simulink model "FreqSweep_HIL"  (Simulink 7.0)
settings: Solver=FixedStepDiscrete  SolverMode=SingleTasking  StartTime=0.0  StopTime=137*20*8*4  FixedStep=1  RelTol=1e-3
InitFcn:
  | %% DSPBuilder Start
  | alt_dspbuilder_update_model(bdroot)
  | %% DSPBuilder End
libraries: allblocks_alteradspbuilder2 x5, simulink x1
settings Model: Creator=lkong  LastModifiedBy=lkong
settings DataIOCC: SignalLoggingName=sigsOut
settings OptimizationCC: InlineInvariantSignals=on
settings DebuggingCC: SaveWithParameterizedLinksMsg=none  SignalResolutionControl=TryResolveAllWithWarning  SolverPrmCheckMsg=none  MultiTaskDSMMsg=warning  MultiTaskCondExecSysMsg=none  StrictBusMsg=None
settings HardwareCC: TargetUnknown=on
settings RTWCC: IncludeERTFirstTime=on
settings GRTTargetCC: TargetFcnLib=ansi_tfl_tmw.mat

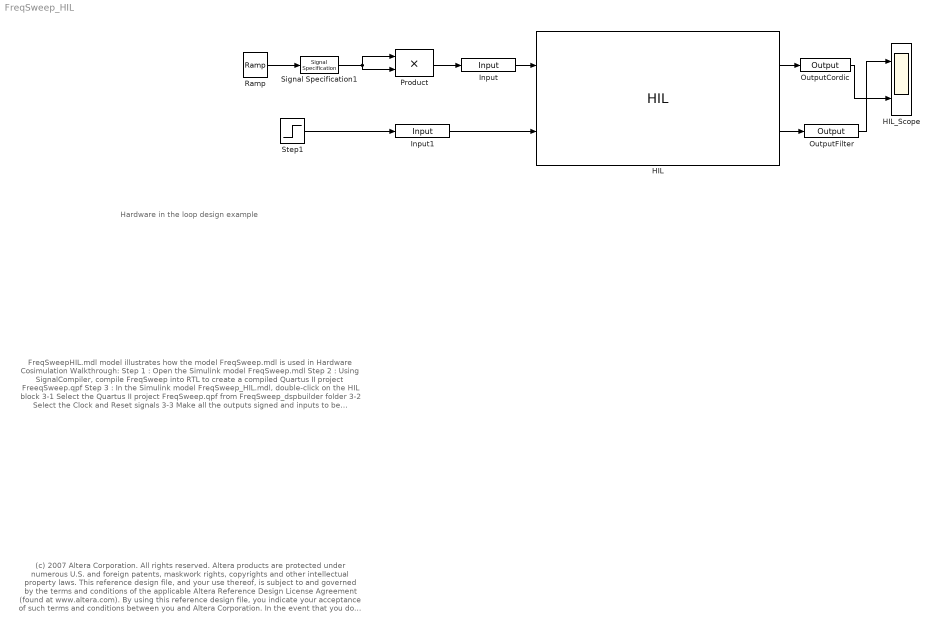
== system FreqSweep_HIL ==
  note: (c) 2007 Altera Corporation. All rights reserved.  Altera products are protected under numerous U.S. and foreign patents, maskwork rights, copyrights and other intellectual property laws.
      | This reference design file, and your use thereof, is subject to and governed by the terms and conditions of the applicable Altera Reference Design License Agreement (found at www.altera.com).
      | By using this reference design file, you indicate your acceptance of such terms and conditions between you and Altera Corporation.
      | In the event that you do not agree with such terms and conditions, you may not use the reference design file and please promptly destroy any copies you have made.
      | This reference design file being provided on an "as-is" basis and as an accommodation and therefore all warranties, representations or guarantees of any kind (whether express, implied or statutory)
      | including, without limitation, warranties of merchantability, non-infringement, or fitness for a particular purpose, are specifically disclaimed.
      | By making this reference design file available, Altera expressly does not recommend, suggest or require that this reference design file be used in combination with any other product not provided by Altera
  note: Hardware in the loop design example
  note: FreqSweepHIL.mdl model illustrates how the model FreqSweep.mdl is used in Hardware Cosimulation
      |
      | Walkthrough:
      | Step 1 : Open the Simulink model FreqSweep.mdl
      | Step 2 : Using SignalCompiler, compile FreqSweep into RTL to create a compiled Quartus II project FreeqSweep.qpf
      | Step 3 : In the Simulink model FreqSweep_HIL.mdl, double-click on the HIL block
      |               3-1 Select the Quartus II project FreqSweep.qpf from FreqSweep_dspbuilder folder
      |               3-2 Select the Clock and Reset signals
      |               3-3 Make all the outputs signed and inputs to be unsigned
      |               3-4 Select the reset active level to match the settings in the original model
      |               3-5 Click on Next to go to page 2 of 2
      |               3-6 Enter the FPGA device value
      |               3-7 Compile with Quartus II
      |               3-8 Scan JTAG and select the JTAG cable
      |               3-9 Program the FPGA on board
      |               3-10 Close the HIL dialog box
      |
      | Step 4 : Simulate in Simulink
  HIL : allblocks_alteradspbuilder2/HIL  entityName=FreqSweep_HIL/HIL  inNames=Input Input1  inBwls="21   1   1   1"  inBwrs="0  0  0  0"  inTypes=u u  inDelayed="1  1"  outNames=OutputCordic OutputFilter  outBwls="21  30"  outBwrs="0  0"  outTypes=s s  resetNames=aclr  InputCount=4  InputNames=Input Clock Input1 aclr  InputWidth="21   1   1   1"  InputRepresentation="0  0  0  0"  InputExport="0  2  0  3"  InputFPP="0  0  0  0"  OutputCount=2  OutputNames=OutputCordic OutputFilter  OutputWidth="21  30"  OutputRepresentation="1  1"  OutputExport="0  0"  OutputFPP="0  0"  JtagCable=3  JtagDevice=1  BurstMode=on  BurstLength=1024  FrameMode=off  SOP=1  OutValid=1  QuartusProject=D:\workspace\Documentation\DesignExamples\Tutorials\HIL\FreqSweep\FreqSweep_dspbuilder\FreqSweep.qpf  HilNewConfig=off  ClockPinLocation=K17  ClockPinSource=0  HilDeviceOnBoard=EP2S60F1020C5  DR_length=56  dspbuilder_reset=on  SLD_NODE_INFO=9622468  AssertSclrBeforeSimulation=1  SampleTime=-1  dspb_ver=5.1  ResetLevel=Active_High  JtagCableName=USB-Blaster [USB-0]  JtagDeviceName=@1: EP2S60 (0x120930DD)  ClockNames=Clock
  HIL_Scope : Scope  NumInputPorts=2
      settings: TimeRange=90000  YMin=-1.5e+006~-600000  YMax=1e+006~600000  MaxDataPoints=15000  Decimation=20
  Input : allblocks_alteradspbuilder2/Input  iofile=d:\p4DspbStd81\P4ws\dsp_builder2\Documentation\DesignExamples\Tutorials\HIL\FreqSweep\tb_FreqSweep_HIL\FreqSweep%5FHIL_Input.salt  BusType=Unsigned Integer  bwl=21  bwr=0  SpecifyClock=off  PORTTYPE=Input  externalType=Inferred  allowFloatingPointOverride=on  logOutputs=off
  Input1 : allblocks_alteradspbuilder2/Input  iofile=d:\p4DspbStd81\P4ws\dsp_builder2\Documentation\DesignExamples\Tutorials\HIL\FreqSweep\tb_FreqSweep_HIL\FreqSweep%5FHIL_Input1.salt  BusType=Single Bit  bwl=1  bwr=0  SpecifyClock=off  PORTTYPE=Input  externalType=Inferred  allowFloatingPointOverride=on  logOutputs=off
  OutputCordic : allblocks_alteradspbuilder2/Output  iofile=d:\p4DspbStd81\P4ws\dsp_builder2\Documentation\DesignExamples\Tutorials\HIL\FreqSweep\tb_FreqSweep_HIL\FreqSweep%5FHIL_OutputCordic.capture  BusType=Signed Integer  bwl=21  bwr=0  externalType=Inferred  PORTTYPE=Output  allowFloatingPointOverride=on  logOutputs=off
  OutputFilter : allblocks_alteradspbuilder2/Output  iofile=d:\p4DspbStd81\P4ws\dsp_builder2\Documentation\DesignExamples\Tutorials\HIL\FreqSweep\tb_FreqSweep_HIL\FreqSweep%5FHIL_OutputFilter.capture  BusType=Signed Integer  bwl=30  bwr=0  externalType=Inferred  PORTTYPE=Output  allowFloatingPointOverride=on  logOutputs=off
  Product : Product  OutDataType=sfix(16)  OutScaling=2^0  SaturateOnIntegerOverflow=on
  Ramp : simulink/Sources/Ramp  SystemSampleTime=-1  slope=.01  start=0  X0=0
  Signal Specification1 : SignalSpecification  SampleTime=1  OutDataType=sfix(16)  OutScaling=2^0
  Step1 : Step  SampleTime=1
  wires:
  Ramp/1 -> Signal Specification1/1
  Signal Specification1/1 -> Product/1, Product/2
  Product/1 -> Input/1
  Step1/1 -> Input1/1
  HIL/1 -> OutputCordic/1
  HIL/2 -> OutputFilter/1
  OutputFilter/1 -> HIL_Scope/1
  OutputCordic/1 -> HIL_Scope/2
  Input1/1 -> HIL/2
  Input/1 -> HIL/1
